simulink subsystem "Day3_Scenario_1"  (R2024a)
settings: Solver=VariableStepAuto  StartTime=0.0  StopTime=10.0  RelTol=1e-3
undefined symbols (not defined in the file): left_first_line_point_x, right_first_line_point_x
libraries: CarMaker4SL x6, slpidlib x1
settings Model: Creator=junhyung.cha  LastModifiedBy=User

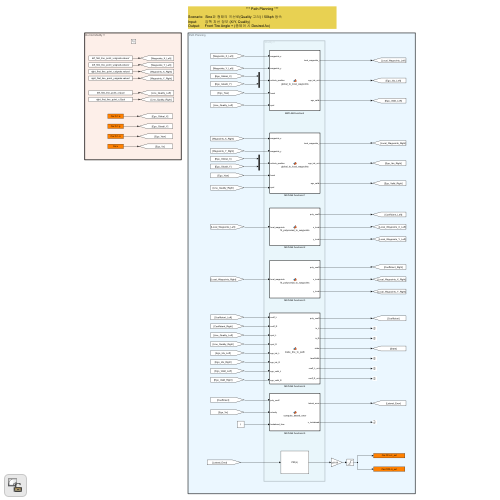
[thumbnail: Simulink's stored preview of the top-level diagram]
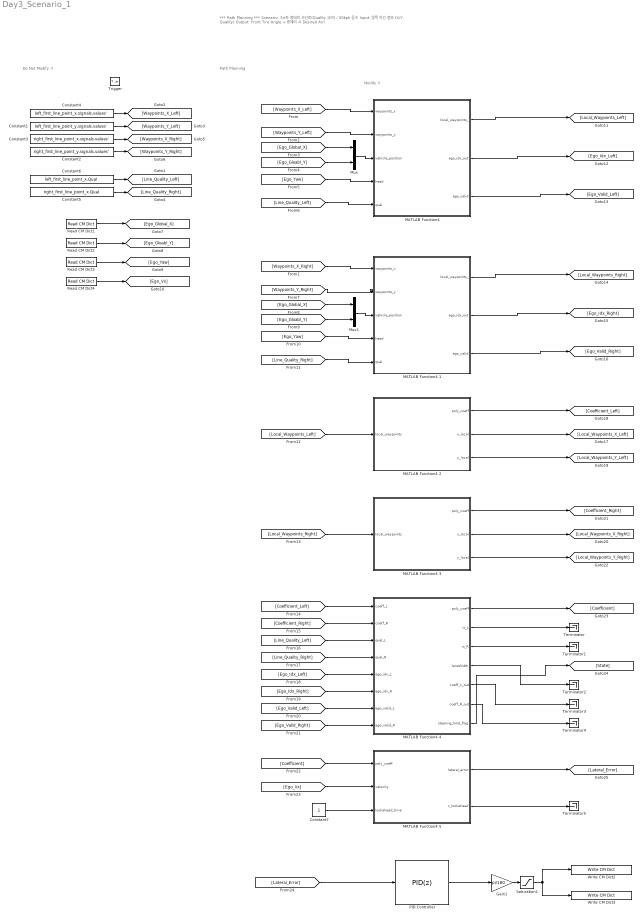
== system Day3_Scenario_1 ==
  note: Path Planning
  note: Do Not Modify !!
  note: Modify !!
  note: *** Path Planning ***
      |
      | Scenario: Sine파 형태의 곡선로(Quality 고려) / 50kph 등속
      | Input: 양쪽 차선 정보 (X/Y, Quality)
      | Output: Front Tire Angle + (종제어 시 Desired Ax)
  Trigger : TriggerPort  TriggerType=function-call  VariantControl=(inherit)
  Constant1 : Constant  Value=left_first_line_point_y.signals.values'
  Constant2 : Constant  Value=right_first_line_point_y.signals.values'
  Constant3 : Constant  Value=right_first_line_point_x.signals.values'
  Constant4 : Constant  Value=left_first_line_point_x.signals.values'
  Constant5 : Constant  Value=right_first_line_point_x.Qual
  Constant6 : Constant  Value=left_first_line_point_x.Qual
  Constant7 : Constant
  Gain1 : Gain  Gain=pi/180
  "MATLAB Function4 " : MATLAB Function  TreatAsAtomicUnit=on
  MATLAB Function4 1 : MATLAB Function  TreatAsAtomicUnit=on
  MATLAB Function4 2 : MATLAB Function  TreatAsAtomicUnit=on
  MATLAB Function4 3 : MATLAB Function  TreatAsAtomicUnit=on
  MATLAB Function4 4 : MATLAB Function  TreatAsAtomicUnit=on
  MATLAB Function4 5 : MATLAB Function  TreatAsAtomicUnit=on
  Mux : Mux  Inputs=2
  Mux1 : Mux  Inputs=2
  PID Controller : slpidlib/PID Controller  Controller=PID  Form=Parallel  TimeDomain=Discrete-time  UseExternalTs=off  SampleTime=-1  IntegratorMethod=Forward Euler  FilterMethod=Forward Euler  ControllerParametersSource=internal  P=2  I=0  UseKiTs=off  D=0  UseExternalDerivativeSource=off  N=100  UseFilter=off  TunerSelectOption=Transfer Function Based (PID Tuner App)  InitialConditionSource=internal  InitialConditionForIntegrator=0  InitialConditionForFilter=0  DifferentiatorICPrevScaledInput=0  ExternalReset=none  TrackingMode=off  Kt=1  LimitOutput=off  SatLimitsSource=internal  UpperSaturationLimit=inf  LowerSaturationLimit=-inf  LinearizeAsGain=on  AntiWindupMode=none  Kb=1  LimitIntegrator=off  UpperIntegratorSaturationLimit=inf  LowerIntegratorSaturationLimit=-inf  POutMin=[]  POutMax=[]  IOutMin=[]  IOutMax=[]  DOutMin=[]  DOutMax=[]  NOutMin=[]  NOutMax=[]  SumOutMin=[]  SumOutMax=[]  SaturationOutMin=[]  SaturationOutMax=[]  PParamMin=[]  PParamMax=[]  IParamMin=[]  IParamMax=[]  DParamMin=[]  DParamMax=[]  NParamMin=[]  NParamMax=[]  KbParamMin=[]  KbParamMax=[]  KtParamMin=[]  KtParamMax=[]  KbOutMin=[]  KbOutMax=[]  KtOutMin=[]  KtOutMax=[]  IntegratorOutMin=[]  IntegratorOutMax=[]  FilterOutMin=[]  FilterOutMax=[]  SumI1OutMin=[]  SumI1OutMax=[]  SumI2OutMin=[]  SumI2OutMax=[]  SumI3OutMin=[]  SumI3OutMax=[]  SumI4OutMin=[]  SumI4OutMax=[]  SumDOutMin=[]  SumDOutMax=[]  DifferentiatorOutMin=[]  DifferentiatorOutMax=[]  FilterDiffOutCoefMin=[]  FilterDiffOutCoefMax=[]  ReciprocalOutMin=[]  ReciprocalOutMax=[]  SumDenOutMin=[]  SumDenOutMax=[]  SumNumOutMin=[]  SumNumOutMax=[]  DivideOutMin=[]  DivideOutMax=[]  UdiffTsProdOutMin=[]  UdiffTsProdOutMax=[]  NTsProdOutMin=[]  NTsProdOutMax=[]  UintegralTsProdOutMin=[]  UintegralTsProdOutMax=[]  UngainTsProdOutMin=[]  UngainTsProdOutMax=[]  ClampingZeroOutDataTypeStr=Inherit: Inherit via back propagation  ClampingZeroOutMin=[]  ClampingZeroOutMax=[]  FilterDenConstantOutDataTypeStr=Inherit: Inherit via back propagation  FilterDenConstantOutMin=[]  FilterDenConstantOutMax=[]  PCopyOutDataTypeStr=Inherit: Inherit via back propagation  PCopyOutMin=[]  PCopyOutMax=[]  NCopyOutDataTypeStr=Inherit: Inherit via back propagation  NCopyOutMin=[]  NCopyOutMax=[]  IntegratorContinuousStateAttributes=''  IntegratorStateMustResolveToSignalObject=off  IntegratorRTWStateStorageClass=Auto  FilterContinuousStateAttributes=''  FilterStateMustResolveToSignalObject=off  FilterRTWStateStorageClass=Auto  ParallelPVariant=InternalParameters  IdealPVariant=Disabled  IVariant=InternalParameters  DVariant=InternalParameters  IntegratorVariant=Discrete  SatVariant=Disabled  AWVariant=Passthrough  PCopyVariant=Disabled  TRVariant=Disabled  FdbkBlocksVariant=Forward  IdealPFdbkVariant=Disabled  SatFdbkVariant=Disabled  DerivativeFilterVariant=Differentiator  NVariant=Passthrough  NCopyVariant=Disabled_SignalSpec  FilterICVariant=InternalICsDifferentiator  IntegratorICVariant=InternalICs  ExternalResetVariant=Disabled  TRSumVariant=Passthrough  SumFdbkVariant=Disabled  SumVariant=Sum_PID  TsampFilterVariant=InternalTs  TsampNgainVariant=Passthrough  TsampIntegralVariant=Disabled_SignalSpec  ExternalSaturationOutDataTypeStr=Inherit: Same as second input  DerivativeSourceVariant=ErrorSignal
  Read CM Dict1 : CarMaker4SL/Read CM Dict  xname=Car.Fr1.tx  xsync=off  xstime=Inherited
  Read CM Dict2 : CarMaker4SL/Read CM Dict  xname=Car.Fr1.ty  xsync=off  xstime=Inherited
  Read CM Dict3 : CarMaker4SL/Read CM Dict  xname=Car.Fr1.rz  xsync=off  xstime=Inherited
  Read CM Dict4 : CarMaker4SL/Read CM Dict  xname=Car.v  xsync=off  xstime=Inherited
  Saturation1 : Saturate  UpperLimit=2  LowerLimit=-2
  Terminator{,1..5} (6 alike) : Terminator
  Write CM Dict2 : CarMaker4SL/Write CM Dict  xname=Car.CFL.rz_ext  xsync=off
  Write CM Dict3 : CarMaker4SL/Write CM Dict  xname=Car.CFR.rz_ext  xsync=off
  wires:
  Constant4/1 -> [Waypoints_X_Left]
  Constant1/1 -> [Waypoints_Y_Left]
  Constant2/1 -> [Waypoints_Y_Right]
  Constant3/1 -> [Waypoints_X_Right]
  [Waypoints_X_Left] -> "MATLAB Function4 "/1(waypoints_x)
  [Waypoints_Y_Left] -> "MATLAB Function4 "/2(waypoints_y)
  Mux/1 -> "MATLAB Function4 "/3(vehicle_position)
  [Ego_Global_X] -> Mux/1
  Read CM Dict2/1 -> [Ego_Gloabl_Y]
  Read CM Dict1/1 -> [Ego_Global_X]
  [Ego_Gloabl_Y] -> Mux/2
  Read CM Dict3/1 -> [Ego_Yaw]
  [Ego_Yaw] -> "MATLAB Function4 "/4(head)
  Constant5/1 -> [Line_Quality_Right]
  Constant6/1 -> [Line_Quality_Left]
  [Line_Quality_Left] -> "MATLAB Function4 "/5(qual)
  [Line_Quality_Right] -> MATLAB Function4 1/5(qual)
  [Ego_Yaw] -> MATLAB Function4 1/4(head)
  [Ego_Gloabl_Y] -> Mux1/2
  [Ego_Global_X] -> Mux1/1
  [Waypoints_Y_Right] -> MATLAB Function4 1/2(waypoints_y)
  [Waypoints_X_Right] -> MATLAB Function4 1/1(waypoints_x)
  Mux1/1 -> MATLAB Function4 1/3(vehicle_position)
  "MATLAB Function4 "/3(ego_valid) -> [Ego_Valid_Left]
  "MATLAB Function4 "/2(ego_idx_out) -> [Ego_Idx_Left]
  "MATLAB Function4 "/1(local_waypoints_) -> [Local_Waypoints_Left]
  MATLAB Function4 1/1(local_waypoints_) -> [Local_Waypoints_Right]
  MATLAB Function4 1/2(ego_idx_out) -> [Ego_Idx_Right]
  MATLAB Function4 1/3(ego_valid) -> [Ego_Valid_Right]
  [Local_Waypoints_Left] -> MATLAB Function4 2/1(local_waypoints)
  [Local_Waypoints_Right] -> MATLAB Function4 3/1(local_waypoints)
  MATLAB Function4 2/1(poly_coeff) -> [Coefficient_Left]
  MATLAB Function4 2/2(x_local) -> [Local_Waypoints_X_Left]
  MATLAB Function4 2/3(y_local) -> [Local_Waypoints_Y_Left]
  MATLAB Function4 3/3(y_local) -> [Local_Waypoints_Y_Right]
  MATLAB Function4 3/2(x_local) -> [Local_Waypoints_X_Right]
  MATLAB Function4 3/1(poly_coeff) -> [Coefficient_Right]
  [Coefficient_Left] -> MATLAB Function4 4/1(coeff_L)
  [Coefficient_Right] -> MATLAB Function4 4/2(coeff_R)
  [Line_Quality_Left] -> MATLAB Function4 4/3(qual_L)
  [Line_Quality_Right] -> MATLAB Function4 4/4(qual_R)
  [Ego_Idx_Left] -> MATLAB Function4 4/5(ego_idx_L)
  [Ego_Idx_Right] -> MATLAB Function4 4/6(ego_idx_R)
  [Ego_Valid_Left] -> MATLAB Function4 4/7(ego_valid_L)
  [Ego_Valid_Right] -> MATLAB Function4 4/8(ego_valid_R)
  MATLAB Function4 4/1(poly_coeff) -> [Coefficient]
  MATLAB Function4 4/7(steering_hold_flag) -> [State]
  MATLAB Function4 4/2(is_L) -> Terminator/1
  MATLAB Function4 4/3(is_R) -> Terminator1/1
  MATLAB Function4 4/5(coeff_L_out) -> Terminator3/1
  MATLAB Function4 4/4(laneWidth) -> Terminator2/1
  MATLAB Function4 4/6(coeff_R_out) -> Terminator4/1
  [Coefficient] -> MATLAB Function4 5/1(poly_coeff)
  Read CM Dict4/1 -> [Ego_Vx]
  [Ego_Vx] -> MATLAB Function4 5/2(velocity)
  Constant7/1 -> MATLAB Function4 5/3(lookahead_time)
  Saturation1/1 -> Write CM Dict3/1, Write CM Dict2/1
  Gain1/1 -> Saturation1/1
  MATLAB Function4 5/1(lateral_error) -> [Lateral_Error]
  MATLAB Function4 5/2(x_lookahead) -> Terminator5/1
  [Lateral_Error] -> PID Controller/1
  PID Controller/1 -> Gain1/1

== matlab function Day3_Scenario_1/MATLAB Function4  ==
  settings: sampleTime=0.1
  data: waypoints_x input; local_waypoints_ output; ego_idx_out output; ego_valid output; waypoints_y input; vehicle_position input; head input; qual input
function [local_waypoints_, ego_idx_out, ego_valid] = global_to_local_waypoints_right( ...
    waypoints_x, waypoints_y, vehicle_position, head, qual)

    % 설정
    N = numel(waypoints_x);
    max_distance = 10;           % 최대 유효 거리 (m)
    lookahead_check_offset = 10; % 앞쪽 quality 확인 길이

    % 출력 초기화
    local_waypoints_ = nan(N, 2);

    % 회전 행렬 파라미터 (차량 heading 기준)
    cos_h = cos(head);
    sin_h = sin(head);

    % 1) 전역 → 로컬 좌표 (qual이 유효한 포인트만 변환)
    for i = 1:N
        if qual(i) == 1
            dx = waypoints_x(i) - vehicle_position(1);
            dy = waypoints_y(i) - vehicle_position(2);
            x_local =  dx * cos_h + dy * sin_h;
            y_local = -dx * sin_h + dy * cos_h;
            local_waypoints_(i, :) = [x_local, y_local];
        end
    end

    % 2) 미래까지 qual이 유지되는 포인트만 true
    forward_valid = false(N, 1);
    for i = 1:N - lookahead_check_offset
        if qual(i) == 1 && all(qual(i:i+lookahead_check_offset) == 1)
            forward_valid(i) = true;
        end
    end

    % 3) 전방 유효 포인트 중 x_local 기준 거리 계산
    x_vals = local_waypoints_(:, 1);
    d_vals = abs(x_vals);

    % forward_valid 크기 맞추기 (뒤쪽 부족한 부분은 false로 유지됨)
    valid_mask = forward_valid & (x_vals >= 0) & (d_vals <= max_distance);

    d_vals(~valid_mask) = Inf;

    % 4) 최소 거리 인덱스 찾기
    [~, ego_idx_out] = min(d_vals);
    if isinf(d_vals(ego_idx_out))
        ego_idx_out = -1;
        ego_valid = 0;
    else
        ego_valid = 1;
    end
end

== matlab function Day3_Scenario_1/MATLAB Function4 1 ==
  settings: sampleTime=0.1
  data: waypoints_x input; local_waypoints_ output; ego_idx_out output; ego_valid output; waypoints_y input; vehicle_position input; head input; qual input
function [local_waypoints_, ego_idx_out, ego_valid] = global_to_local_waypoints_right( ...
    waypoints_x, waypoints_y, vehicle_position, head, qual)

    % 설정
    N = numel(waypoints_x);
    max_distance = 10;           % 최대 유효 거리 (m)
    lookahead_check_offset = 10; % 앞쪽 quality 확인 길이

    % 출력 초기화
    local_waypoints_ = nan(N, 2);

    % 회전 행렬 파라미터 (차량 heading 기준)
    cos_h = cos(head);
    sin_h = sin(head);

    % 1) 전역 → 로컬 좌표 (qual이 유효한 포인트만 변환)
    for i = 1:N
        if qual(i) == 1
            dx = waypoints_x(i) - vehicle_position(1);
            dy = waypoints_y(i) - vehicle_position(2);
            x_local =  dx * cos_h + dy * sin_h;
            y_local = -dx * sin_h + dy * cos_h;
            local_waypoints_(i, :) = [x_local, y_local];
        end
    end

    % 2) 미래까지 qual이 유지되는 포인트만 true
    forward_valid = false(N, 1);
    for i = 1:N - lookahead_check_offset
        if qual(i) == 1 && all(qual(i:i+lookahead_check_offset) == 1)
            forward_valid(i) = true;
        end
    end

    % 3) 전방 유효 포인트 중 x_local 기준 거리 계산
    x_vals = local_waypoints_(:, 1);
    d_vals = abs(x_vals);

    % forward_valid 크기 맞추기 (뒤쪽 부족한 부분은 false로 유지됨)
    valid_mask = forward_valid & (x_vals >= 0) & (d_vals <= max_distance);

    d_vals(~valid_mask) = Inf;

    % 4) 최소 거리 인덱스 찾기
    [~, ego_idx_out] = min(d_vals);
    if isinf(d_vals(ego_idx_out))
        ego_idx_out = -1;
        ego_valid = 0;
    else
        ego_valid = 1;
    end
end

== matlab function Day3_Scenario_1/MATLAB Function4 2 ==
  settings: sampleTime=0.1
  data: local_waypoints input; poly_coeff output; x_local output; y_local output
function [poly_coeff, x_local, y_local] = fit_polynomial_to_waypoints(local_waypoints)
%#codegen
% Sliding-Window 기반 3차 다항식 피팅 (예외 및 이상치 핸들링 추가)
% local_waypoints : Nx2 [x y] in vehicle-local frame
% poly_coeff      : 1x4 [a3 a2 a1 a0]
% x_local, y_local: MAX_POINTS×1 윈도우에 저장된 값 (나머지는 0)

    %% 파라미터
    MAX_DIST      = 13.0;    % 전방 최대 거리 [m]
    MAX_POINTS    = 10;      % 최대 포인트 개수
    POLY_ORDER    = 3;       % 3차 다항식 차수
    COEFF_LIMIT   = 100;     % 계수 이상치 기준 (절대값)

    %% 이전 경로 계수 저장용
    persistent prev_poly_coeff;
    if isempty(prev_poly_coeff)
        prev_poly_coeff = zeros(1, POLY_ORDER+1);
    end

    %% 출력 초기화
    poly_coeff = prev_poly_coeff;  % 기본은 이전 경로 유지
    x_local    = zeros(MAX_POINTS,1);
    y_local    = zeros(MAX_POINTS,1);

    %% 슬라이딩 윈도우에 실제 저장된 점 개수
    stored = 0;
    x_all = local_waypoints(:,1);
    y_all = local_waypoints(:,2);

    %% 1) 전방 필터링 + 윈도우 저장
    for i = 1:length(x_all)
        if x_all(i) > 0 && x_all(i) < MAX_DIST
            if stored < MAX_POINTS
                stored = stored + 1;
                x_local(stored) = x_all(i);
                y_local(stored) = y_all(i);
            end
        end
    end

    %% 2) 충분한 점이 있을 때만 피팅, 이상치 핸들링
    if stored >= (POLY_ORDER + 1)
        % 다항식 피팅
        coeff = polyfit(x_local(1:stored), y_local(1:stored), POLY_ORDER);
        % 계수 유효성 검사: 유한성 및 제한값 내부 여부
        if all(isfinite(coeff)) && all(abs(coeff) < COEFF_LIMIT)
            poly_coeff = coeff;
            prev_poly_coeff = coeff;  % 상태 갱신
        else
            % 피팅 결과 이상치 발생 시 이전 경로 유지
            poly_coeff = prev_poly_coeff;
        end
    end
end

== matlab function Day3_Scenario_1/MATLAB Function4 3 ==
  settings: sampleTime=0.1
  data: local_waypoints input; poly_coeff output; x_local output; y_local output
function [poly_coeff, x_local, y_local] = fit_polynomial_to_waypoints(local_waypoints)
%#codegen
% Sliding-Window 기반 3차 다항식 피팅 (예외 및 이상치 핸들링 추가)
% local_waypoints : Nx2 [x y] in vehicle-local frame
% poly_coeff      : 1x4 [a3 a2 a1 a0]
% x_local, y_local: MAX_POINTS×1 윈도우에 저장된 값 (나머지는 0)

    %% 파라미터
    MAX_DIST      = 13.0;    % 전방 최대 거리 [m]
    MAX_POINTS    = 10;      % 최대 포인트 개수
    POLY_ORDER    = 3;       % 3차 다항식 차수
    COEFF_LIMIT   = 100;     % 계수 이상치 기준 (절대값)

    %% 이전 경로 계수 저장용
    persistent prev_poly_coeff;
    if isempty(prev_poly_coeff)
        prev_poly_coeff = zeros(1, POLY_ORDER+1);
    end

    %% 출력 초기화
    poly_coeff = prev_poly_coeff;  % 기본은 이전 경로 유지
    x_local    = zeros(MAX_POINTS,1);
    y_local    = zeros(MAX_POINTS,1);

    %% 슬라이딩 윈도우에 실제 저장된 점 개수
    stored = 0;
    x_all = local_waypoints(:,1);
    y_all = local_waypoints(:,2);

    %% 1) 전방 필터링 + 윈도우 저장
    for i = 1:length(x_all)
        if x_all(i) > 0 && x_all(i) < MAX_DIST
            if stored < MAX_POINTS
                stored = stored + 1;
                x_local(stored) = x_all(i);
                y_local(stored) = y_all(i);
            end
        end
    end

    %% 2) 충분한 점이 있을 때만 피팅, 이상치 핸들링
    if stored >= (POLY_ORDER + 1)
        % 다항식 피팅
        coeff = polyfit(x_local(1:stored), y_local(1:stored), POLY_ORDER);
        % 계수 유효성 검사: 유한성 및 제한값 내부 여부
        if all(isfinite(coeff)) && all(abs(coeff) < COEFF_LIMIT)
            poly_coeff = coeff;
            prev_poly_coeff = coeff;  % 상태 갱신
        else
            % 피팅 결과 이상치 발생 시 이전 경로 유지
            poly_coeff = prev_poly_coeff;
        end
    end
end

== matlab function Day3_Scenario_1/MATLAB Function4 4 ==
  settings: sampleTime=0.1
  data: coeff_L input; poly_coeff output; is_L output; is_R output; laneWidth output; coeff_L_out output; coeff_R_out output; coeff_R input; qual_L input; qual_R input; ego_idx_L input; ego_idx_R input; ego_valid_L input; ego_valid_R input; steering_hold_flag output
function [poly_coeff, is_L, is_R, laneWidth, coeff_L_out, coeff_R_out, steering_hold_flag] = make_line_to_path( ...
    coeff_L, coeff_R, qual_L, qual_R, ego_idx_L, ego_idx_R, ego_valid_L, ego_valid_R)
%#codegen
persistent Lw prev_coeff_path
if isempty(Lw) || isempty(prev_coeff_path)
    Lw = 3.5;
    prev_coeff_path = zeros(1,4);
end

% 1) 좌/우 차선 유효성 판정 (최소 5포인트)
is_L = sum(qual_L) >= 5;
is_R = sum(qual_R) >= 5;

% 2) 양쪽 다 인식되면 차폭 갱신
if is_L && is_R
    x_mid = linspace(0,30,20);
    yL = polyval(coeff_L, x_mid);
    yR = polyval(coeff_R, x_mid);
    valid = isfinite(yL) & isfinite(yR);
    if nnz(valid) >= 3
        w = abs(yR(valid) - yL(valid));
        mw = mean(w);
        if mw >= 2 && mw <= 5
            Lw = 0.9 * Lw + 0.1 * mw;
        end
    end
end

% 차폭 최소값 보장
Lw = max(Lw, 2.5);
halfW = Lw / 2;

% 초기화
steering_hold_flag = 0;

% 3) 경로 결정
if is_L && is_R
    if ego_valid_L && ego_valid_R && ego_idx_L > 0 && ego_idx_R > 0
        % 가까운 쪽 차선에 더 비중 두어 중심선 결정
        wL = 1 / ego_idx_L;
        wR = 1 / ego_idx_R;
        sumW = wL + wR;
        alpha = wL / sumW;
        poly_coeff = alpha * coeff_R + (1 - alpha) * coeff_L;
    else
        % 두 차선은 있지만 ego 인덱스 없음 → 조향 홀드
        poly_coeff = prev_coeff_path;
        steering_hold_flag = 1;
    end

elseif is_L
    poly_coeff = coeff_L;
    poly_coeff(end) = poly_coeff(end) - halfW;

elseif is_R
    poly_coeff = coeff_R;
    poly_coeff(end) = poly_coeff(end) + halfW;

else
    % 둘 다 차선 없음 → 이전 경로 유지 + 조향 홀드
    poly_coeff = prev_coeff_path;
    steering_hold_flag = 1;
end

% 4) 상태 갱신
laneWidth = Lw;
coeff_L_out = coeff_L;
coeff_R_out = coeff_R;
prev_coeff_path = poly_coeff;
end

== matlab function Day3_Scenario_1/MATLAB Function4 5 ==
  settings: sampleTime=0.1
  data: poly_coeff input; lateral_error output; x_lookahead output; velocity input; lookahead_time input
function [lateral_error, x_lookahead] = compute_lateral_error(poly_coeff, velocity, lookahead_time)
%#codegen
% compute_lateral_error - Look-ahead 지점에서의 lateral error 계산
%   poly_coeff     : 1x4 다항식 계수 [a3 a2 a1 a0]
%   velocity       : 차량 전진 속도 (m/s)
%   lookahead_time : look-ahead 시간 (s)
%
% 출력:
%   lateral_error  : lateral error + heading error 보정값
%   x_lookahead    : look-ahead 거리

    %% 1) lookahead 거리
    x_lookahead = velocity * lookahead_time;

    %% 2) 경로상의 y 위치
    y = polyval(poly_coeff, x_lookahead);

    %% 3) 경로 기울기 → 방향 각도
    dpoly = polyder(poly_coeff);
    dy_dx = polyval(dpoly, x_lookahead);
    path_theta = atan(dy_dx);

    %% 4) heading error (차량 방향 θ_vehicle = 0 가정)
    heading_error = path_theta;

    %% 5) lateral error 보정 (tunable gain)
    k_heading = 1.0;  
    lateral_error = y + k_heading * heading_error;
    
end
